simulink model "MainSim"  (R2025a)
settings: Solver=VariableStepAuto  StartTime=0.0  StopTime=110  MaxStep=0.01  RelTol=1e-3
undefined symbols (not defined in the file): bref, cref, g, inertia, m, m_carriage
libraries: fl_lib x79, nesl_utility x32, simulink_extras x9, sdl_lib x4, aerolibobsolete x2, ee_lib x2, slpidlib x2, aerolibadyn x1, matrix_library x1, aerolibatmos2 x1, aerolibwind2 x1, aerolibanim x1
(part 3 of 5)

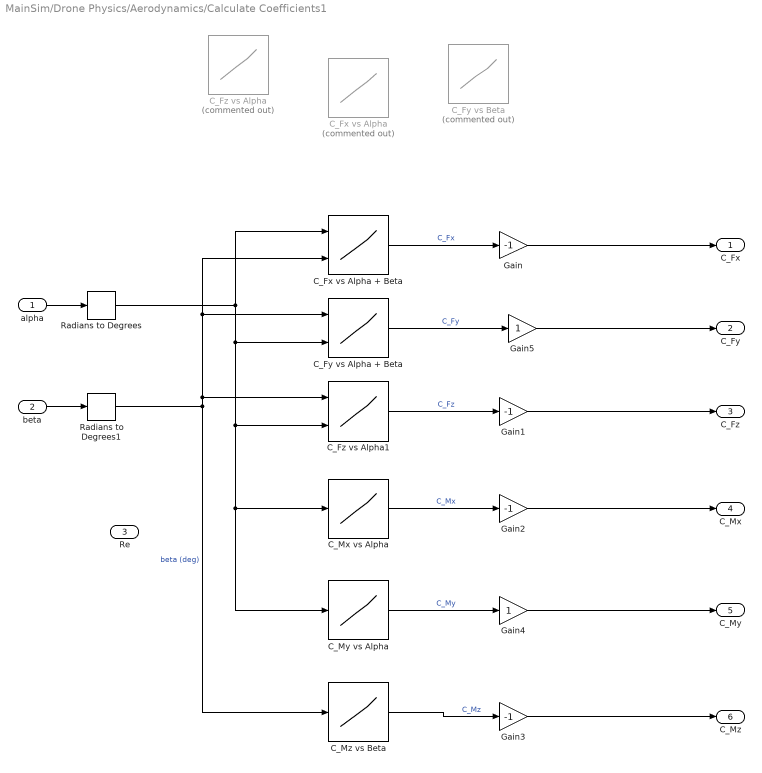
== system MainSim/Drone Physics/Aerodynamics/Calculate Coefficients1 ==
  alpha : Inport
  beta : Inport  Port=2
  Re : Inport  Port=3
  C_Fx vs Alpha : Lookup_n-D  Commented=on  NumberOfTableDimensions=1  BreakpointsForDimension1=[-30;-24;-18;-12;-6;-1;1;6;12;18;24;30]  Table=[-0.8477543;-0.5413928;-0.2881651;-0.0989454;0.01802407;0.06513188;0.06513188;0.01802407;-0.0989454;-0.2881651;-0.5413928;-0.8477543]  InternalRulePriority=Speed  RndMeth=Simplest
  C_Fx vs Alpha + Beta : Lookup_n-D  BreakpointsForDimension1=[-20;-18;-16;-14;-12;-10;-8;-6;-4;-2;0;2;4;6;8;10;12;14;16;18;20]  BreakpointsForDimension2=[-20;-18;-16;-14;-12;-10;-8;-6;-4;-2;0;2;4;6;8;10;12;14;16;18;20]  Table=[-0.614358525 -0.552468628 -0.496975921 -0.447963654 -0.405402727 -0.369395384 -0.339949206 -0.317050883 -0.300725231 -0.290929286 -0.287706806 -0.290929286 -0.300725231 -0.317050883 -0.339949206 -0.369395384 -0.405402727 -0.447963654 -0.496975921 -0.552468628 -0.614358525;-0.551607695 -0.489072561 -0.432947474 -0.383480964 -0.340566675 -0.304256004 -0.274532451 -0.251406615 -0.234924884 -0.22504748 -0.221789714 -0.22504748 -0.234924884 -0.251406615 -0.274532451 -0.304256004 -0.340566675 -0.383480964 -0.432947474 -0.489072561 -0.551607695;-0.495317375 -0.432168752 -0.375672546 -0.325789814 -0.282533426 -0.245910781 -0.215944692 -0.192643052 -0.176018972 -0.16606146 -0.162782923 -0.16606146 -0.176018972 -0.192643052 -0.215944692 -0.245910781 -0.282533426 -0.325789814 -0.375672546 -0.432168752 -0.495317375;-0.445552671 -0.382005906 -0.325091967 -0.274839973 -0.231277677 -0.194399013 -0.164233169 -0.140770136 -0.124023873 -0.113987385 -0.110686666 -0.113987385 -0.124023873 -0.140770136 -0.164233169 -0.194399013 -0.231277677 -0.274839973 -0.325091967 -0.382005906 -0.445552671;-0.40242558 -0.338476077 -0.281206427 -0.230652283 -0.186829361 -0.149732411 -0.119392246 -0.095788054 -0.07893594700000001 -0.06885042800000001 -0.065514827 -0.06885042800000001 -0.07893594700000001 -0.095788054 -0.119392246 -0.149732411 -0.186829361 -0.230652283 -0.281206427 -0.338476077 -0.40242558;-0.365919483 -0.301631518 -0.244075562 -0.193256152 -0.149204048 -0.111925303 -0.081432692 -0.057717714 -0.040804565 -0.030673395 -0.027308541 -0.030673395 -0.040804565 -0.057717714 -0.081432692 -0.111925303 -0.149204048 -0.193256152 -0.244075562 -0.301631518 -0.365919483;-0.336041187 -0.271485221 -0.213680187 -0.162651643 -0.118419577 -0.080997789 -0.050375282 -0.026586135 -0.009594434000000001 0.000582762 0.003952354 0.000582762 -0.009594434000000001 -0.026586135 -0.050375282 -0.080997789 -0.118419577 -0.162651643 -0.213680187 -0.271485221 -0.336041187;-0.312780091 -0.248011918 -0.190027999 -0.138840895 -0.094478059 -0.056945223 -0.026238136 -0.00236637 0.014675995 0.024884562 0.028280614 0.024884562 0.014675995 -0.00236637 -0.026238136 -0.056945223 -0.094478059 -0.138840895 -0.190027999 -0.248011918 -0.312780091;-0.296181899 -0.231254063 -0.173135414 -0.121838779 -0.077382601 -0.039773232 -0.008997109 0.014930056 0.032010963 0.042247716 0.045634461 0.042247716 0.032010963 0.014930056 -0.008997109 -0.039773232 -0.077382601 -0.121838779 -0.173135414 -0.231254063 -0.296181899;-0.28623251 -0.221218221 -0.163015263 -0.11165277 -0.06713633400000001 -0.029480985 0.001340551 0.025308445 0.042403284 0.052657162 0.0560561 0.052657162 0.042403284 0.025308445 0.001340551 -0.029480985 -0.06713633400000001 -0.11165277 -0.163015263 -0.221218221 -0.28623251;-0.217886618 -0.217886618 -0.15966593 -0.108275856 -0.06373363 -0.026060496 0.004776964 0.028752083 0.045865859 0.056122123 0.059524976 0.056122123 0.045865859 0.028752083 0.004776964 -0.026060496 -0.06373363 -0.108275856 -0.15966593 -0.217886618 -0.217886618;-0.28623251 -0.221218221 -0.163015263 -0.11165277 -0.06713633400000001 -0.029480985 0.001340551 0.025308445 0.042403284 0.052657162 0.0560561 0.052657162 0.042403284 0.025308445 0.001340551 -0.029480985 -0.06713633400000001 -0.11165277 -0.163015263 -0.221218221 -0.28623251;-0.296181899 -0.231254063 -0.173135414 -0.121838779 -0.077382601 -0.039773232 -0.008997109 0.014930056 0.032010963 0.042247716 0.045634461 0.042247716 0.032010963 0.014930056 -0.008997109 -0.039773232 -0.077382601 -0.121838779 -0.173135414 -0.231254063 -0.296181899;-0.312780091 -0.248011918 -0.190027999 -0.138840895 -0.094478059 -0.056945223 -0.026238136 -0.00236637 0.014675995 0.024884562 0.028280614 0.024884562 0.014675995 -0.00236637 -0.026238136 -0.056945223 -0.094478059 -0.138840895 -0.190027999 -0.248011918 -0.312780091;-0.336041187 -0.271485221 -0.213680187 -0.162651643 -0.118419577 -0.080997789 -0.050375282 -0.026586135 -0.009594434000000001 0.000582762 0.003952354 0.000582762 ...(+1790 chars)]  InternalRulePriority=Speed  RndMeth=Simplest
      settings: InputPortMap=u0,u1
  C_Fy vs Alpha + Beta : Lookup_n-D  BreakpointsForDimension1=[-20;-18;-16;-14;-12;-10;-8;-6;-4;-2;0;2;4;6;8;10;12;14;16;18;20]  BreakpointsForDimension2=[-20;-18;-16;-14;-12;-10;-8;-6;-4;-2;0;2;4;6;8;10;12;14;16;18;20]  Table=[1.66195002 1.66627986 1.67002882 1.67327787 1.67699593 1.67878935 1.68047312 1.6822726 1.68322903 1.68369328 1.68391417 1.68369328 1.68322903 1.6822726 1.68047312 1.67878935 1.67699593 1.67327787 1.67002882 1.66627986 1.66195002;1.50492698 1.50889275 1.51325693 1.51613012 1.5186286 1.52053747 1.52211226 1.5230983 1.52411176 1.52465096 1.52475781 1.52465096 1.52411176 1.5230983 1.52211226 1.52053747 1.5186286 1.51613012 1.51325693 1.50889275 1.50492698;1.3449861 1.34965961 1.35276007 1.3553714 1.35760143 1.35922371 1.36072185 1.36169609 1.36221375 1.36277715 1.36305841 1.36277715 1.36221375 1.36169609 1.36072185 1.35922371 1.35760143 1.3553714 1.35276007 1.34965961 1.3449861;1.18364169 1.18651461 1.18940186 1.1919222 1.19406535 1.19564439 1.19670122 1.1974075 1.19789162 1.19833631 1.19861313 1.19833631 1.19789162 1.1974075 1.19670122 1.19564439 1.19406535 1.1919222 1.18940186 1.18651461 1.18364169;1.01863302 1.02137777 1.02382367 1.02623563 1.02802096 1.0291959 1.03039533 1.03091195 1.03143754 1.03171442 1.03166744 1.03171442 1.03143754 1.03091195 1.03039533 1.0291959 1.02802096 1.02623563 1.02382367 1.02137777 1.01863302;0.85160149 0.854263182 0.856389587 0.85839774 0.860011937 0.861116685 0.8621121899999999 0.862633629 0.862917173 0.863469112 0.863402469 0.863469112 0.862917173 0.862633629 0.8621121899999999 0.861116685 0.860011937 0.85839774 0.856389587 0.854263182 0.85160149;0.683145201 0.6854003870000001 0.687448977 0.689359965 0.690391124 0.691442623 0.691573132 0.692106162 0.69270664 0.693189344 0.693075696 0.693189344 0.69270664 0.692106162 0.691573132 0.691442623 0.690391124 0.689359965 0.687448977 0.6854003870000001 0.683145201;0.513680454 0.515516389 0.51700176 0.518329265 0.519440831 0.520452311 0.51978407 0.520476755 0.521151285 0.521719227 0.521682795 0.521719227 0.521151285 0.520476755 0.51978407 0.520452311 0.519440831 0.518329265 0.51700176 0.515516389 0.513680454;0.342987019 0.344595797 0.345799223 0.346543215 0.347632555 0.346986164 0.34735697 0.34791355 0.348772052 0.349005705 0.348832678 0.349005705 0.348772052 0.34791355 0.34735697 0.346986164 0.347632555 0.346543215 0.345799223 0.344595797 0.342987019;0.171657723 0.172615507 0.173702671 0.174327657 0.174967248 0.1739672 0.1742629 0.174639945 0.175310283 0.175362274 0.175197751 0.175362274 0.175310283 0.174639945 0.1742629 0.1739672 0.174967248 0.174327657 0.173702671 0.172615507 0.171657723;-0.000932729 -0.000932729 -0.001325927 -0.001861466 -0.002017838 -0.000728378 -0.000836194 -0.001162275 -0.00131784 -0.001113439 -0.00023498 -0.001113439 -0.00131784 -0.001162275 -0.000836194 -0.000728378 -0.002017838 -0.001861466 -0.001325927 -0.000932729 -0.000932729;-0.171657723 -0.172615507 -0.173702671 -0.174327657 -0.174967248 -0.1739672 -0.1742629 -0.174639945 -0.175310283 -0.175362274 -0.175197751 -0.175362274 -0.175310283 -0.174639945 -0.1742629 -0.1739672 -0.174967248 -0.174327657 -0.173702671 -0.172615507 -0.171657723;-0.342987019 -0.344595797 -0.345799223 -0.346543215 -0.347632555 -0.346986164 -0.34735697 -0.34791355 -0.348772052 -0.349005705 -0.348832678 -0.349005705 -0.348772052 -0.34791355 -0.34735697 -0.346986164 -0.347632555 -0.346543215 -0.345799223 -0.344595797 -0.342987019;-0.513680454 -0.515516389 -0.51700176 -0.518329265 -0.519440831 -0.520452311 -0.51978407 -0.520476755 -0.521151285 -0.521719227 -0.521682795 -0.521719227 -0.521151285 -0.520476755 -0.51978407 -0.520452311 -0.519440831 -0.518329265 -0.51700176 -0.515516389 -0.513680454;-0.683145201 -0.6854003870000001 -0.687448977 -0.689359965 -0.690391124 -0.691442623 -0.691573132 -0.692106162 -0.69270664 -0.693189344 -0.693075696 -0.693189344 -0.69270664 -0.692106162 -0.691573132 -0.691442623 -0.690391124 -0.689359965 -0.687448977 -0.6854003870000001 -0.683145201;-0.85160149 -0.854263182 -0.856389587 -0.85839774 -0.860011937 -0.861116685 -0.8621121899999999 -0.862633629 -0.862917173 -0.863469112 -0.863402469 -0.863469112 -0.862917173 -0.862633629 -0.8621121899999999 -0.861116685 -0.860011937 ...(+1294 chars)]  ExtrapMethod=Clip  InternalRulePriority=Speed  RndMeth=Simplest
      settings: InputPortMap=u0,u1
  C_Fy vs Beta : Lookup_n-D  Commented=on  NumberOfTableDimensions=1  BreakpointsForDimension1=[-30;-24;-18;-12;-6;-1;1;6;12;16;20;25;30;35;40;45;50;60;70;90]  Table=[-2.6204513;-2.2457427000000001;-1.7747444000000001;-1.2274444;-0.62725549999999997;-0.079830300000000007;0.079830310000000002;0.62725547000000004;1.22744436;1.6399999999999999;1.8999999999999999;1.1000000000000001;1.05;1;1;1;0.90000000000000002;0.5;0.29999999999999999;0]  ExtrapMethod=Clip  InternalRulePriority=Speed  RndMeth=Simplest
  C_Fz vs Alpha : Lookup_n-D  Commented=on  NumberOfTableDimensions=1  BreakpointsForDimension1=[-30;-24;-18;-12;-6;-1;1;6;12;16;20;25;30;35;40;45;50;60;70;90]  Table=[-2.6204513;-2.2457427000000001;-1.7747444000000001;-1.2274444;-0.62725549999999997;-0.079830300000000007;0.079830310000000002;0.62725547000000004;1.22744436;1.6399999999999999;1.8999999999999999;1.1000000000000001;1.05;1;1;1;0.90000000000000002;0.5;0.29999999999999999;0]  ExtrapMethod=Clip  InternalRulePriority=Speed  RndMeth=Simplest
  C_Fz vs Alpha1 : Lookup_n-D  BreakpointsForDimension1=[-20;-18;-16;-14;-12;-10;-8;-6;-4;-2;0;2;4;6;8;10;12;14;16;18;20]  BreakpointsForDimension2=[-20;-18;-16;-14;-12;-10;-8;-6;-4;-2;0;2;4;6;8;10;12;14;16;18;20]  Table=[-1.55009948 -1.40370092 -1.25462317 -1.10283778 -0.949156016 -0.7935119390000001 -0.636432656 -0.477775325 -0.318386645 -0.158573043 -0.001764467 0.158573043 0.318386645 0.477775325 0.636432656 0.7935119390000001 0.949156016 1.10283778 1.25462317 1.40370092 1.55009948;-1.57242746 -1.42392316 -1.27291412 -1.11875403 -0.962481446 -0.804477256 -0.644911779 -0.484281407 -0.322789156 -0.160769242 -0.002307224 0.160769242 0.322789156 0.484281407 0.644911779 0.804477256 0.962481446 1.11875403 1.27291412 1.42392316 1.57242746;-1.59261224 -1.44260011 -1.28893724 -1.13291699 -0.974830801 -0.814870303 -0.653020572 -0.490346781 -0.32667547 -0.162246361 -0.002565448 0.162246361 0.32667547 0.490346781 0.653020572 0.814870303 0.974830801 1.13291699 1.28893724 1.44260011 1.59261224;-1.61091112 -1.45846414 -1.30317135 -1.14538593 -0.985506982 -0.823595326 -0.660151009 -0.495668672 -0.330141696 -0.163784707 -0.002650902 0.163784707 0.330141696 0.495668672 0.660151009 0.823595326 0.985506982 1.14538593 1.30317135 1.45846414 1.61091112;-1.62580438 -1.47213576 -1.31538824 -1.15589718 -0.994589284 -0.831455457 -0.666675567 -0.500644752 -0.333363011 -0.165359101 -0.002762659 0.165359101 0.333363011 0.500644752 0.666675567 0.831455457 0.994589284 1.15589718 1.31538824 1.47213576 1.62580438;-1.6394278 -1.48424315 -1.32634589 -1.16560392 -1.00278587 -0.838339093 -0.672240555 -0.50496377 -0.33688758 -0.167824235 -0.002242482 0.167824235 0.33688758 0.50496377 0.672240555 0.838339093 1.00278587 1.16560392 1.32634589 1.48424315 1.6394278;-1.65045554 -1.49444956 -1.33532388 -1.17333149 -1.00982805 -0.844082802 -0.677467162 -0.509090802 -0.339530444 -0.169133362 -0.001356052 0.169133362 0.339530444 0.509090802 0.677467162 0.844082802 1.00982805 1.17333149 1.33532388 1.49444956 1.65045554;-1.65862927 -1.50181487 -1.34209337 -1.1796587 -1.01530082 -0.84885035 -0.681215192 -0.5120618220000001 -0.341559843 -0.170311443 -0.00127523 0.170311443 0.341559843 0.5120618220000001 0.681215192 0.84885035 1.01530082 1.1796587 1.34209337 1.50181487 1.65862927;-1.66490423 -1.507349 -1.34699511 -1.18436577 -1.01945538 -0.853198533 -0.684158833 -0.514192369 -0.343166457 -0.17152109 -0.000870461 0.17152109 0.343166457 0.514192369 0.684158833 0.853198533 1.01945538 1.18436577 1.34699511 1.507349 1.66490423;-1.66880981 -1.51086475 -1.35022719 -1.18731356 -1.02212124 -0.855586551 -0.686012383 -0.515670089 -0.344273714 -0.172312963 -0.000435662 0.172312963 0.344273714 0.515670089 0.686012383 0.855586551 1.02212124 1.18731356 1.35022719 1.51086475 1.66880981;-1.5118782 -1.5118782 -1.35139134 -1.18847636 -1.02316789 -0.856422645 -0.686794229 -0.516544166 -0.344670939 -0.172784026 -4.74e-05 0.172784026 0.344670939 0.516544166 0.686794229 0.856422645 1.02316789 1.18847636 1.35139134 1.5118782 1.5118782;-1.66880981 -1.51086475 -1.35022719 -1.18731356 -1.02212124 -0.855586551 -0.686012383 -0.515670089 -0.344273714 -0.172312963 -0.000435662 0.172312963 0.344273714 0.515670089 0.686012383 0.855586551 1.02212124 1.18731356 1.35022719 1.51086475 1.66880981;-1.66490423 -1.507349 -1.34699511 -1.18436577 -1.01945538 -0.853198533 -0.684158833 -0.514192369 -0.343166457 -0.17152109 -0.000870461 0.17152109 0.343166457 0.514192369 0.684158833 0.853198533 1.01945538 1.18436577 1.34699511 1.507349 1.66490423;-1.65862927 -1.50181487 -1.34209337 -1.1796587 -1.01530082 -0.84885035 -0.681215192 -0.5120618220000001 -0.341559843 -0.170311443 -0.00127523 0.170311443 0.341559843 0.5120618220000001 0.681215192 0.84885035 1.01530082 1.1796587 1.34209337 1.50181487 1.65862927;-1.65045554 -1.49444956 -1.33532388 -1.17333149 -1.00982805 -0.844082802 -0.677467162 -0.509090802 -0.339530444 -0.169133362 -0.001356052 0.169133362 0.339530444 0.509090802 0.677467162 0.844082802 1.00982805 1.17333149 1.33532388 1.49444956 1.65045554;-1.6394278 -1.48424315 -1.32634589 -1.16560392 -1.00278587 -0.838339093 -0.672240555 -0.50496377 -0.33688758 -0.167824235 -0.002242482 0.167824235 0.33688758 0.50496377 0.672240555 ...(+1353 chars)]  ExtrapMethod=Clip  InternalRulePriority=Speed  RndMeth=Simplest
      settings: InputPortMap=u0,u1
  C_Mx vs Alpha : Lookup_n-D  NumberOfTableDimensions=1  BreakpointsForDimension1=[-15;-11.25;-7.5;-3.75;-2;-1.7777780000000001;-1.5555559999999999;-1.3333330000000001;-1.111111;-0.88888900000000004;-0.66666700000000001;-0.44444400000000001;-0.222222;0;0.222222;0.44444400000000001;0.66666700000000001;0.88888900000000004;1.111111;1.3333330000000001;1.5555559999999999;1.7777780000000001;2;3.75;7.5;11.25;15]  Table=[8.330000000000001e-05;4.3e-05;1.83e-05;3.47e-06;5.9e-07;3.8e-07;2.58e-07;1.93e-07;1.74e-07;1.53e-07;1.57e-07;2e-07;2.8e-07;-3.94e-07;-2.8e-07;-2e-07;-1.57e-07;-1.53e-07;-1.74e-07;-1.93e-07;-2.58e-07;-3.8e-07;-5.9e-07;-3.47e-06;-1.83e-05;-4.3e-05;-8.330000000000001e-05]  InternalRulePriority=Speed  RndMeth=Simplest
  C_My vs Alpha : Lookup_n-D  NumberOfTableDimensions=1  BreakpointsForDimension1=[-30;-24;-18;-12;-6;-1;1;6;12;18;24;30]  Table=[0.63433291;0.54398872;0.43026972;0.29781773;0.15227498;0.01398048;-0.0139805;-0.152275;-0.2978177;-0.4302697;-0.5439887;-0.6343329]  InternalRulePriority=Speed  RndMeth=Simplest
  C_Mz vs Beta : Lookup_n-D  NumberOfTableDimensions=1  BreakpointsForDimension1=[-30;-24;-18;-12;-6;-1;1;6;12;18;24;30]  Table=[0.63433291;0.54398872;0.43026972;0.29781773;0.15227498;0.01398048;-0.0139805;-0.152275;-0.2978177;-0.4302697;-0.5439887;-0.6343329]  InternalRulePriority=Speed  RndMeth=Simplest
  Gain{,1..3} (4 alike) : Gain  Gain=-1
  Gain4 : Gain
  Gain5 : Gain
  Radians to Degrees : simulink_extras/Transformations/Radians to Degrees
  Radians to Degrees1 : simulink_extras/Transformations/Radians to Degrees
  C_Fx : Outport
  C_Fy : Outport  Port=2
  C_Fz : Outport  Port=3
  C_Mx : Outport  Port=4
  C_My : Outport  Port=5
  C_Mz : Outport  Port=6
  wires:
  Gain5/1 -> C_Fy/1
  Gain4/1 -> C_My/1
  Gain3/1 -> C_Mz/1
  Gain2/1 -> C_Mx/1
  Gain1/1 -> C_Fz/1
  Gain/1 -> C_Fx/1
  Radians to Degrees1/1 -> C_Fz vs Alpha1/1, C_Fy vs Alpha + Beta/1, C_Fx vs Alpha + Beta/2, C_Mz vs Beta/1  "beta (deg)"
  Radians to Degrees/1 -> C_Fx vs Alpha + Beta/1, C_Fy vs Alpha + Beta/2, C_Fz vs Alpha1/2, C_Mx vs Alpha/1, C_My vs Alpha/1
  C_Mz vs Beta/1 -> Gain3/1  "C_Mz"
  C_My vs Alpha/1 -> Gain4/1  "C_My"
  C_Mx vs Alpha/1 -> Gain2/1  "C_Mx"
  beta/1 -> Radians to Degrees1/1
  alpha/1 -> Radians to Degrees/1
  C_Fy vs Alpha + Beta/1 -> Gain5/1  "C_Fy"
  C_Fz vs Alpha1/1 -> Gain1/1  "C_Fz"
  C_Fx vs Alpha + Beta/1 -> Gain/1  "C_Fx"

== system MainSim/Drone Physics/EoM/Combine Forces & Moments ==
  Aerodynamics : Inport
  Gravity : Inport  Port=2
  Propulsion : Inport  Port=3
  CG : Inport  Port=4
  Add : Sum  Inputs=+++
  Add1 : Sum  Inputs=++++++
  Bus Selector : BusSelector  OutputSignals=F_B,M_B,S_B
  Bus Selector1 : BusSelector  OutputSignals=F_B,M_B,S_B
  Bus Selector2 : BusSelector  OutputSignals=F_B,M_B
  Cross Product : matrix_library/Cross Product
  Gain : Gain  Gain=1/cref
  Subtract : Sum  Inputs=+-
  Terminator : Terminator
  F_B' : Outport
  M_B' : Outport  Port=2
  wires:
  Aerodynamics/1 -> Bus Selector/1
  Gravity/1 -> Bus Selector1/1
  Add/1 -> F_B'/1  "F_B'"
  Add1/1 -> M_B'/1
  Bus Selector/1 -> Cross Product/2, Add/1  "<F_B>"
  Bus Selector1/1 -> Add/2  "<F_B>"
  Bus Selector/2 -> Add1/1  "<M_B>"
  Bus Selector/3 -> Subtract/1  "<S_B>"
  Subtract/1 -> Cross Product/1
  Cross Product/1 -> Add1/2
  Gain/1 -> Terminator/1  "CG/C"
  CG/1 -> Gain/1, Subtract/2
  Propulsion/1 -> Bus Selector2/1
  Bus Selector2/2 -> Add1/3  "<M_B>"
  Bus Selector2/1 -> Add/3  "<F_B>"

== system MainSim/Drone Physics/EoM/Direction Cosine Matrix Calculation ==
  Eul_BL : Inport
  Demux : Demux  Outputs=3
  Ground : Ground
  Rotation Angles to Direction Cosine Matrix : Angle2Dcm
      settings: AttributesFormatString=Rotation Order: %<rotationOrder>
  Terminator : Terminator
  Terminator1 : Terminator
  Transpose : Math  Operator=transpose
  Vector Concatenate : Concatenate  NumInputs=3
  DCM_B'B : Outport
  DCM_BB' : Outport  Port=2
  wires:
  Demux/3 -> Terminator1/1
  Transpose/1 -> DCM_B'B/1  "DCM_B'B"
  Vector Concatenate/1 -> Rotation Angles to Direction Cosine Matrix/1
  Rotation Angles to Direction Cosine Matrix/1 -> DCM_BB'/1, Transpose/1  "DCM_BB'"
  Ground/1 -> Vector Concatenate/2, Vector Concatenate/1
  Demux/2 -> Terminator/1
  Demux/1 -> Vector Concatenate/3
  Eul_BL/1 -> Demux/1

== system MainSim/Drone Physics/EoM/Ground Detect Trigger - Termination ==
  X_BE_E : Inport
  Ground Level : Constant  Value=ground_level
  Relational Operator : RelationalOperator  Operator=>  OutDataTypeStr=boolean  RndMeth=Simplest  InputSameDT=off
  Selector : Selector  InputPortWidth=3  IndexOptions=Index vector (dialog)  Indices=[3]  OutputSizes=1
  Stop Simulation : Stop
  wires:
  Relational Operator/1 -> Stop Simulation/1
  Ground Level/1 -> Relational Operator/2
  X_BE_E/1 -> Selector/1
  Selector/1 -> Relational Operator/1

== system MainSim/Drone Physics/EoM/Running Avg ==
  u : Inport
  MATLAB Function : MATLAB Function  TreatAsAtomicUnit=on
  Out1 : Outport
  wires:
  u/1 -> MATLAB Function/1(u)
  MATLAB Function/1(y) -> Out1/1

== system MainSim/Drone Physics/EoM/Running Avg1 ==
  u : Inport
  MATLAB Function : MATLAB Function  TreatAsAtomicUnit=on
  Out1 : Outport
  wires:
  u/1 -> MATLAB Function/1(u)
  MATLAB Function/1(y) -> Out1/1

== system MainSim/Drone Physics/EoM/Running Avg2 ==
  u : Inport
  MATLAB Function : MATLAB Function  TreatAsAtomicUnit=on
  Out1 : Outport
  wires:
  u/1 -> MATLAB Function/1(u)
  MATLAB Function/1(y) -> Out1/1

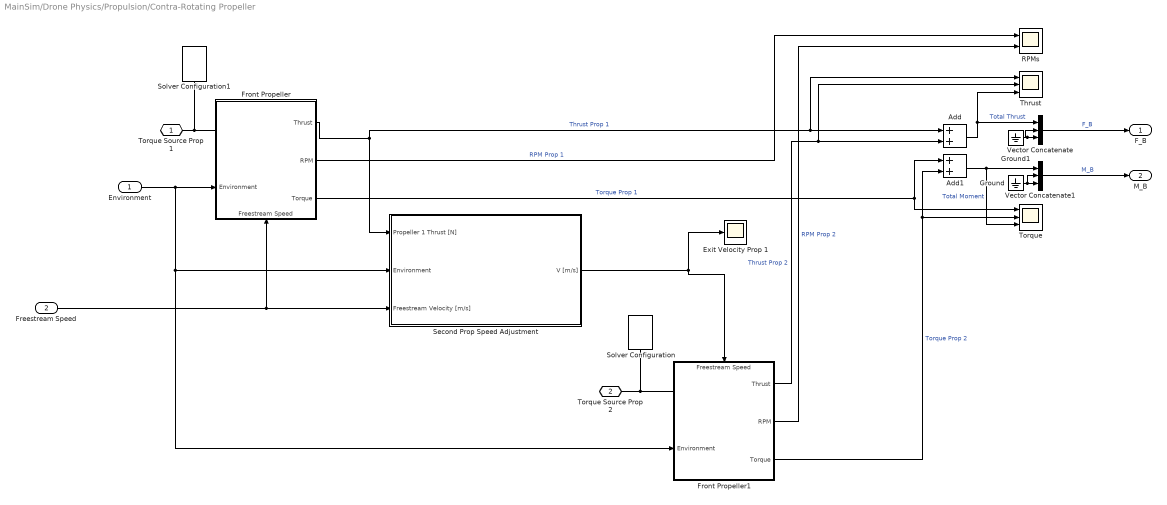
== system MainSim/Drone Physics/Propulsion/Contra-Rotating Propeller ==
  Environment : Inport
  Freestream Speed : Inport  Port=2
  Add : Sum
  Add1 : Sum
  Exit Velocity Prop 1 : Scope
      settings: ActiveDisplayYMinimum=-0.56468572092452329  ActiveDisplayYMaximum=5.0821714883207108  DataLoggingVariableName=ScopeData5
  Front Propeller : Subsystem
      settings: PortSchema="{\"entries\":[{\"content\":{\"sides\":[{\"content\":{\"connectorIds\":[\"LConn1\",\"In1\"]},\"type\":\"ConnectorPlacement.EquallySpacedRectSide\",\"uuid\":\"73d37dfa-c503-43f9-9596-b5e45f2bb291\"},{\"content\":{\"connectorIds\":[\"Out1\",\"Out2\",\"Out3\"],\"side\":\"RIGHT\"},\"type\":\"ConnectorPlacement.EquallySpacedRectSide\",\"uuid\":\"3674c389-2fff-4609-bdea-497312b626f0\"},{\"content\":{\"side\":\"TOP\"},\"type\":\"ConnectorPlacement.EquallySpacedRectSide\",\"uuid\":\"4ddff869-abc5-41ea-b654-b1a87db3aebf\"},{\"content\":{\"connectorIds\":[\"In2\"],\"side\":\"BOTTOM\"},\"type\":\"ConnectorPlacement.EquallySpacedRectSide\",\"uuid\":\"b118b9bb-d518-4709-95e5-457ee8be32dc\"}]},\"type\":\"ConnectorPlacement.EquallySpacedConnector\",\"uuid\":\"ef4d0754-f307-49aa-90cb-f59c4d3f0201\"}],\"packageUris\":[\"http://schema.mathworks.com/mf0/Connector/R2020b\"],\"version\":\"1.0\"}"
  Front Propeller1 : Subsystem
      settings: PortSchema="{\"entries\":[{\"content\":{\"sides\":[{\"content\":{\"connectorIds\":[\"LConn1\",\"In1\"]},\"type\":\"ConnectorPlacement.EquallySpacedRectSide\",\"uuid\":\"73d37dfa-c503-43f9-9596-b5e45f2bb291\"},{\"content\":{\"connectorIds\":[\"Out1\",\"Out2\",\"Out3\"],\"side\":\"RIGHT\"},\"type\":\"ConnectorPlacement.EquallySpacedRectSide\",\"uuid\":\"3674c389-2fff-4609-bdea-497312b626f0\"},{\"content\":{\"connectorIds\":[\"In2\"],\"side\":\"TOP\"},\"type\":\"ConnectorPlacement.EquallySpacedRectSide\",\"uuid\":\"4ddff869-abc5-41ea-b654-b1a87db3aebf\"}]},\"type\":\"ConnectorPlacement.EquallySpacedConnector\",\"uuid\":\"ef4d0754-f307-49aa-90cb-f59c4d3f0201\"}],\"packageUris\":[\"http://schema.mathworks.com/mf0/Connector/R2020b\"],\"version\":\"1.0\"}"
  Ground : Ground
  Ground1 : Ground
  RPMs : Scope  NumInputPorts=2
      settings: ActiveDisplayYMinimum=-11573.712044991189  ActiveDisplayYMaximum=11896.938453382989  DataLoggingVariableName=ScopeData4
  Second Prop Speed Adjustment : Subsystem
  Solver Configuration : nesl_utility/Solver Configuration  PhysicalDomain=network_engine_domain  SubClassName=solver  LeftPortType=input  RightPortType=generic  Tones=[]  Harmonics=[]  SimulateNoise=off  Profile=off  UseLocalSampling=off  EnableSwitchedLinearOptims=on  FrequencyDomain=off  UseCCode=off  RelTol=0.001  AbsTol=0.001  MinStep=1e-09  ToWorkspace=off  RevertToSquareIcSolve=off  NumHomotopyIterations=100  PhasorMode=off  PhasorModeNumHarmonics=1  ConsistencySolver=NEWTON_XTOL_AFTER_FTOL  IndexReductionMethod=DerivativeReplacement  DoDC=off  ResidualTolerance=1e-09  ConsistencyTolSource=GLOBAL  ConsistencyAbsTol=0.001  ConsistencyRelTol=0.001  ConsistencyTolFactor=0.001  UseLocalSolver=off  LocalSolverChoice=NE_BACKWARD_EULER_ADVANCER  ResolveIndetEquations=on  FunctionEvalNumThread=1  LocalSolverSampleTime=0.001  DoFixedCost=off  MaxNonlinIter=3  MaxModeIter=2  ComputeImpulses=off  ImpulseIterations=2  LinearAlgebra=auto  LinearAlgebraNumThread=0  EquationFormulation=NE_TIME_EF  DelaysMemoryBudget=1024  AutomaticFiltering=on  FilteringTimeConstant=0.001  PartitionStorageMethod=AS_NEEDED  PartitionMemoryBudget=1024  PartitionMethod=ROBUST  MultibodyUseLocalSolver=off  MultibodyLocalSolverChoice=ODE1  MultibodyLocalSolverSampleTime=0.001
  Solver Configuration1 : nesl_utility/Solver Configuration  PhysicalDomain=network_engine_domain  SubClassName=solver  LeftPortType=input  RightPortType=generic  Tones=[]  Harmonics=[]  SimulateNoise=off  Profile=off  UseLocalSampling=off  EnableSwitchedLinearOptims=on  FrequencyDomain=off  UseCCode=off  RelTol=0.001  AbsTol=0.001  MinStep=1e-09  ToWorkspace=off  RevertToSquareIcSolve=off  NumHomotopyIterations=100  PhasorMode=off  PhasorModeNumHarmonics=1  ConsistencySolver=NEWTON_XTOL_AFTER_FTOL  IndexReductionMethod=DerivativeReplacement  DoDC=off  ResidualTolerance=1e-09  ConsistencyTolSource=GLOBAL  ConsistencyAbsTol=0.001  ConsistencyRelTol=0.001  ConsistencyTolFactor=0.001  UseLocalSolver=off  LocalSolverChoice=NE_BACKWARD_EULER_ADVANCER  ResolveIndetEquations=on  FunctionEvalNumThread=1  LocalSolverSampleTime=0.001  DoFixedCost=off  MaxNonlinIter=3  MaxModeIter=2  ComputeImpulses=off  ImpulseIterations=2  LinearAlgebra=auto  LinearAlgebraNumThread=0  EquationFormulation=NE_TIME_EF  DelaysMemoryBudget=1024  AutomaticFiltering=on  FilteringTimeConstant=0.001  PartitionStorageMethod=AS_NEEDED  PartitionMemoryBudget=1024  PartitionMethod=ROBUST  MultibodyUseLocalSolver=off  MultibodyLocalSolverChoice=ODE1  MultibodyLocalSolverSampleTime=0.001
  Thrust : Scope  NumInputPorts=3
      settings: ActiveDisplayYMinimum=-0.51224883046910774  ActiveDisplayYMaximum=4.1562383451302329
  Torque : Scope  NumInputPorts=3
      settings: ActiveDisplayYMinimum=-0.0788123767098801  ActiveDisplayYMaximum=0.078815374675042418  DataLoggingVariableName=ScopeData6
  Vector Concatenate : Concatenate  NumInputs=3
  Vector Concatenate1 : Concatenate  NumInputs=3
  Torque Source Prop 1 : PMIOPort  Side=Left
  Torque Source Prop 2 : PMIOPort  Port=2  Side=Left
  F_B : Outport
  M_B : Outport  Port=2
  wires:
  Add/1 -> Thrust/3, Vector Concatenate/1  "Total Thrust"
  Freestream Speed/1 -> Front Propeller/2(Freestream Speed), Second Prop Speed Adjustment/3(Freestream Velocity [m/s])
  Ground/1 -> Vector Concatenate1/2, Vector Concatenate1/3
  Vector Concatenate/1 -> F_B/1  "F_B"
  Front Propeller1/1(Thrust) -> Thrust/2, Add/2  "Thrust Prop 2"
  Front Propeller/3(Torque) -> Torque/1, Add1/1  "Torque Prop 1"
  Ground1/1 -> Vector Concatenate/2, Vector Concatenate/3
  Front Propeller1/3(Torque) -> Add1/2, Torque/2  "Torque Prop 2"
  Front Propeller1/2(RPM) -> RPMs/2  "RPM Prop 2"
  Vector Concatenate1/1 -> M_B/1  "M_B"
  Environment/1 -> Front Propeller1/1(Environment), Second Prop Speed Adjustment/2(Environment), Front Propeller/1(Environment)
  Front Propeller/2(RPM) -> RPMs/1  "RPM Prop 1"
  Second Prop Speed Adjustment/1(V [m/s]) -> Front Propeller1/2(Freestream Speed), Exit Velocity Prop 1/1
  Add1/1 -> Torque/3, Vector Concatenate1/1  "Total Moment"
  Front Propeller/1(Thrust) -> Thrust/1, Add/1, Second Prop Speed Adjustment/1(Propeller 1 Thrust [N])  "Thrust Prop 1"
  connections:
  Torque Source Prop 2/RConn1 -- Front Propeller1/LConn1 -- Solver Configuration/RConn1
  Torque Source Prop 1/RConn1 -- Solver Configuration1/RConn1 -- Front Propeller/LConn1

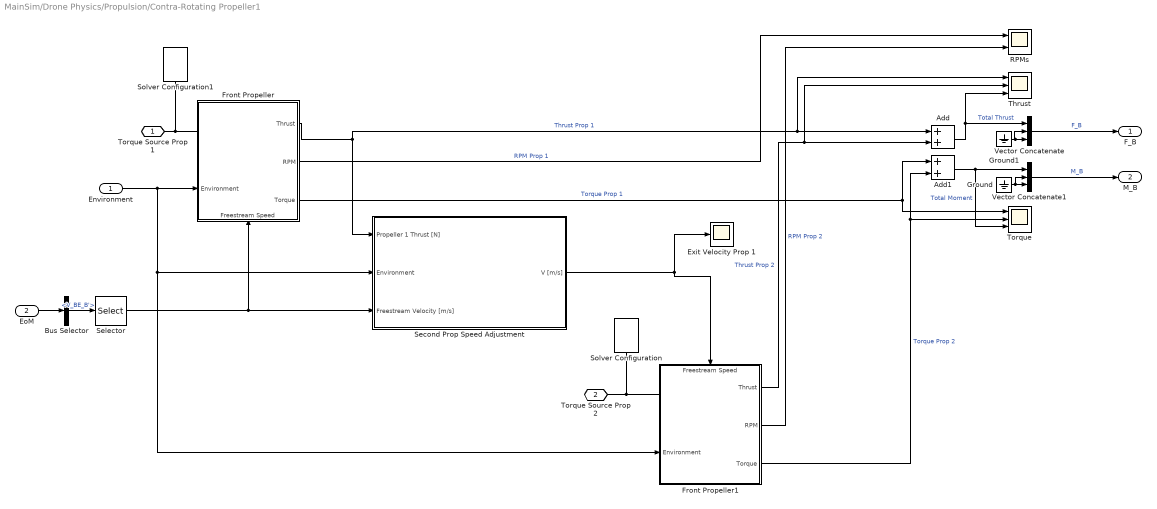
== system MainSim/Drone Physics/Propulsion/Contra-Rotating Propeller1 ==
  Environment : Inport
  EoM : Inport  Port=2
  Add : Sum
  Add1 : Sum
  Bus Selector : BusSelector  OutputSignals=V_BE_B'
  Exit Velocity Prop 1 : Scope
      settings: ActiveDisplayYMinimum=8.9336789456286088  ActiveDisplayYMaximum=11.068772464025542  DataLoggingVariableName=ScopeData5
  Front Propeller : Subsystem
      settings: PortSchema="{\"entries\":[{\"content\":{\"sides\":[{\"content\":{\"connectorIds\":[\"LConn1\",\"In1\"]},\"type\":\"ConnectorPlacement.EquallySpacedRectSide\",\"uuid\":\"73d37dfa-c503-43f9-9596-b5e45f2bb291\"},{\"content\":{\"connectorIds\":[\"Out1\",\"Out2\",\"Out3\"],\"side\":\"RIGHT\"},\"type\":\"ConnectorPlacement.EquallySpacedRectSide\",\"uuid\":\"3674c389-2fff-4609-bdea-497312b626f0\"},{\"content\":{\"side\":\"TOP\"},\"type\":\"ConnectorPlacement.EquallySpacedRectSide\",\"uuid\":\"4ddff869-abc5-41ea-b654-b1a87db3aebf\"},{\"content\":{\"connectorIds\":[\"In2\"],\"side\":\"BOTTOM\"},\"type\":\"ConnectorPlacement.EquallySpacedRectSide\",\"uuid\":\"b118b9bb-d518-4709-95e5-457ee8be32dc\"}]},\"type\":\"ConnectorPlacement.EquallySpacedConnector\",\"uuid\":\"ef4d0754-f307-49aa-90cb-f59c4d3f0201\"}],\"packageUris\":[\"http://schema.mathworks.com/mf0/Connector/R2020b\"],\"version\":\"1.0\"}"
  Front Propeller1 : Subsystem
      settings: PortSchema="{\"entries\":[{\"content\":{\"sides\":[{\"content\":{\"connectorIds\":[\"LConn1\",\"In1\"]},\"type\":\"ConnectorPlacement.EquallySpacedRectSide\",\"uuid\":\"73d37dfa-c503-43f9-9596-b5e45f2bb291\"},{\"content\":{\"connectorIds\":[\"Out1\",\"Out2\",\"Out3\"],\"side\":\"RIGHT\"},\"type\":\"ConnectorPlacement.EquallySpacedRectSide\",\"uuid\":\"3674c389-2fff-4609-bdea-497312b626f0\"},{\"content\":{\"connectorIds\":[\"In2\"],\"side\":\"TOP\"},\"type\":\"ConnectorPlacement.EquallySpacedRectSide\",\"uuid\":\"4ddff869-abc5-41ea-b654-b1a87db3aebf\"}]},\"type\":\"ConnectorPlacement.EquallySpacedConnector\",\"uuid\":\"ef4d0754-f307-49aa-90cb-f59c4d3f0201\"}],\"packageUris\":[\"http://schema.mathworks.com/mf0/Connector/R2020b\"],\"version\":\"1.0\"}"
  Ground : Ground
  Ground1 : Ground
  RPMs : Scope  NumInputPorts=2
      settings: ActiveDisplayYMinimum=-11573.712044991189  ActiveDisplayYMaximum=11896.938453382989  DataLoggingVariableName=ScopeData4
  Second Prop Speed Adjustment : Subsystem
  Selector : Selector  InputPortWidth=3  IndexOptions=Index vector (dialog)  Indices=[1]  OutputSizes=1
  Solver Configuration : nesl_utility/Solver Configuration  PhysicalDomain=network_engine_domain  SubClassName=solver  LeftPortType=input  RightPortType=generic  Tones=[]  Harmonics=[]  SimulateNoise=off  Profile=off  UseLocalSampling=off  EnableSwitchedLinearOptims=on  FrequencyDomain=off  UseCCode=off  RelTol=0.001  AbsTol=0.001  MinStep=1e-09  ToWorkspace=off  RevertToSquareIcSolve=off  NumHomotopyIterations=100  PhasorMode=off  PhasorModeNumHarmonics=1  ConsistencySolver=NEWTON_XTOL_AFTER_FTOL  IndexReductionMethod=DerivativeReplacement  DoDC=off  ResidualTolerance=1e-09  ConsistencyTolSource=GLOBAL  ConsistencyAbsTol=0.001  ConsistencyRelTol=0.001  ConsistencyTolFactor=0.001  UseLocalSolver=off  LocalSolverChoice=NE_BACKWARD_EULER_ADVANCER  ResolveIndetEquations=on  FunctionEvalNumThread=1  LocalSolverSampleTime=0.001  DoFixedCost=off  MaxNonlinIter=3  MaxModeIter=2  ComputeImpulses=off  ImpulseIterations=2  LinearAlgebra=auto  LinearAlgebraNumThread=0  EquationFormulation=NE_TIME_EF  DelaysMemoryBudget=1024  AutomaticFiltering=on  FilteringTimeConstant=0.001  PartitionStorageMethod=AS_NEEDED  PartitionMemoryBudget=1024  PartitionMethod=ROBUST  MultibodyUseLocalSolver=off  MultibodyLocalSolverChoice=ODE1  MultibodyLocalSolverSampleTime=0.001
  Solver Configuration1 : nesl_utility/Solver Configuration  PhysicalDomain=network_engine_domain  SubClassName=solver  LeftPortType=input  RightPortType=generic  Tones=[]  Harmonics=[]  SimulateNoise=off  Profile=off  UseLocalSampling=off  EnableSwitchedLinearOptims=on  FrequencyDomain=off  UseCCode=off  RelTol=0.001  AbsTol=0.001  MinStep=1e-09  ToWorkspace=off  RevertToSquareIcSolve=off  NumHomotopyIterations=100  PhasorMode=off  PhasorModeNumHarmonics=1  ConsistencySolver=NEWTON_XTOL_AFTER_FTOL  IndexReductionMethod=DerivativeReplacement  DoDC=off  ResidualTolerance=1e-09  ConsistencyTolSource=GLOBAL  ConsistencyAbsTol=0.001  ConsistencyRelTol=0.001  ConsistencyTolFactor=0.001  UseLocalSolver=off  LocalSolverChoice=NE_BACKWARD_EULER_ADVANCER  ResolveIndetEquations=on  FunctionEvalNumThread=1  LocalSolverSampleTime=0.001  DoFixedCost=off  MaxNonlinIter=3  MaxModeIter=2  ComputeImpulses=off  ImpulseIterations=2  LinearAlgebra=auto  LinearAlgebraNumThread=0  EquationFormulation=NE_TIME_EF  DelaysMemoryBudget=1024  AutomaticFiltering=on  FilteringTimeConstant=0.001  PartitionStorageMethod=AS_NEEDED  PartitionMemoryBudget=1024  PartitionMethod=ROBUST  MultibodyUseLocalSolver=off  MultibodyLocalSolverChoice=ODE1  MultibodyLocalSolverSampleTime=0.001
  Thrust : Scope  NumInputPorts=3
      settings: ActiveDisplayYMinimum=0.33826860057429142  ActiveDisplayYMaximum=0.39208387213902191
  Torque : Scope  NumInputPorts=3
      settings: ActiveDisplayYMinimum=-0.01855336181218363  ActiveDisplayYMaximum=0.018553497462872586  DataLoggingVariableName=ScopeData6
  Vector Concatenate : Concatenate  NumInputs=3
  Vector Concatenate1 : Concatenate  NumInputs=3
  Torque Source Prop 1 : PMIOPort  Side=Left
  Torque Source Prop 2 : PMIOPort  Port=2  Side=Left
  F_B : Outport
  M_B : Outport  Port=2
  wires:
  Add/1 -> Thrust/3, Vector Concatenate/1  "Total Thrust"
  Selector/1 -> Front Propeller/2(Freestream Speed), Second Prop Speed Adjustment/3(Freestream Velocity [m/s])
  Ground/1 -> Vector Concatenate1/2, Vector Concatenate1/3
  Vector Concatenate/1 -> F_B/1  "F_B"
  Front Propeller1/1(Thrust) -> Thrust/2, Add/2  "Thrust Prop 2"
  Front Propeller/3(Torque) -> Torque/1, Add1/1  "Torque Prop 1"
  Ground1/1 -> Vector Concatenate/2, Vector Concatenate/3
  Front Propeller1/3(Torque) -> Add1/2, Torque/2  "Torque Prop 2"
  Front Propeller1/2(RPM) -> RPMs/2  "RPM Prop 2"
  Vector Concatenate1/1 -> M_B/1  "M_B"
  Environment/1 -> Front Propeller1/1(Environment), Second Prop Speed Adjustment/2(Environment), Front Propeller/1(Environment)
  Front Propeller/2(RPM) -> RPMs/1  "RPM Prop 1"
  Second Prop Speed Adjustment/1(V [m/s]) -> Front Propeller1/2(Freestream Speed), Exit Velocity Prop 1/1
  Add1/1 -> Torque/3, Vector Concatenate1/1  "Total Moment"
  Front Propeller/1(Thrust) -> Thrust/1, Add/1, Second Prop Speed Adjustment/1(Propeller 1 Thrust [N])  "Thrust Prop 1"
  EoM/1 -> Bus Selector/1
  Bus Selector/1 -> Selector/1  "<V_BE_B'>"
  connections:
  Torque Source Prop 2/RConn1 -- Front Propeller1/LConn1 -- Solver Configuration/RConn1
  Torque Source Prop 1/RConn1 -- Solver Configuration1/RConn1 -- Front Propeller/LConn1

== system MainSim/Drone Physics/Propulsion/ESC and Motor ==
  Input Motor 1 : Inport
  Input Motor 2 : Inport  Port=2
  Gain : Gain  Gain=-1
  Gain1 : Gain
  Ideal Angular Velocity Source : fl_lib/Mechanical/Mechanical Sources/Ideal Angular Velocity Source
  Ideal Angular Velocity Source1 : fl_lib/Mechanical/Mechanical Sources/Ideal Angular Velocity Source
  Mechanical Rotational Reference : fl_lib/Mechanical/Rotational Elements/Mechanical Rotational Reference
  Mechanical Rotational Reference1 : fl_lib/Mechanical/Rotational Elements/Mechanical Rotational Reference
  Scope : Scope  NumInputPorts=2
      settings: ActiveDisplayYMinimum=-1  ActiveDisplayYMaximum=1  DataLoggingVariableName=ScopeData11
  Simulink-PS Converter : nesl_utility/Simulink-PS Converter  PhysicalDomain=network_engine_domain  SubClassName=ps_input  LeftPortType=input  RightPortType=output  PseudoPeriodic=off  Frequencies=[]  NoiseDistribution=none  NoiseParameters=[]  Unit=rad/s  AffineConversion=off  FilteringAndDerivatives=filter  SimscapeFilterOrder=1  InputFilterTimeConstant=0.001  UdotUserProvided=0
  Simulink-PS Converter1 : nesl_utility/Simulink-PS Converter  PhysicalDomain=network_engine_domain  SubClassName=ps_input  LeftPortType=input  RightPortType=output  PseudoPeriodic=off  Frequencies=[]  NoiseDistribution=none  NoiseParameters=[]  Unit=rad/s  AffineConversion=off  FilteringAndDerivatives=filter  SimscapeFilterOrder=1  InputFilterTimeConstant=0.001  UdotUserProvided=0
  Transfer Fcn : TransferFcn  Numerator=[1000]  Denominator=[1/20 1]
  Transfer Fcn1 : TransferFcn  Numerator=[1000]  Denominator=[1/20 1]
  Motor 1 : PMIOPort  Side=Right
  Motor 2 : PMIOPort  Port=2  Side=Right
  wires:
  Gain/1 -> Scope/2, Simulink-PS Converter1/1
  Transfer Fcn/1 -> Scope/1, Simulink-PS Converter/1
  Input Motor 2/1 -> Transfer Fcn1/1
  Input Motor 1/1 -> Gain1/1
  Transfer Fcn1/1 -> Gain/1
  Gain1/1 -> Transfer Fcn/1
  connections:
  Ideal Angular Velocity Source1/LConn1 -- Motor 2/RConn1
  Ideal Angular Velocity Source/RConn1 -- Simulink-PS Converter/RConn1
  Ideal Angular Velocity Source/LConn1 -- Motor 1/RConn1
  Mechanical Rotational Reference/LConn1 -- Ideal Angular Velocity Source/RConn2
  Mechanical Rotational Reference1/LConn1 -- Ideal Angular Velocity Source1/RConn2
  Ideal Angular Velocity Source1/RConn1 -- Simulink-PS Converter1/RConn1

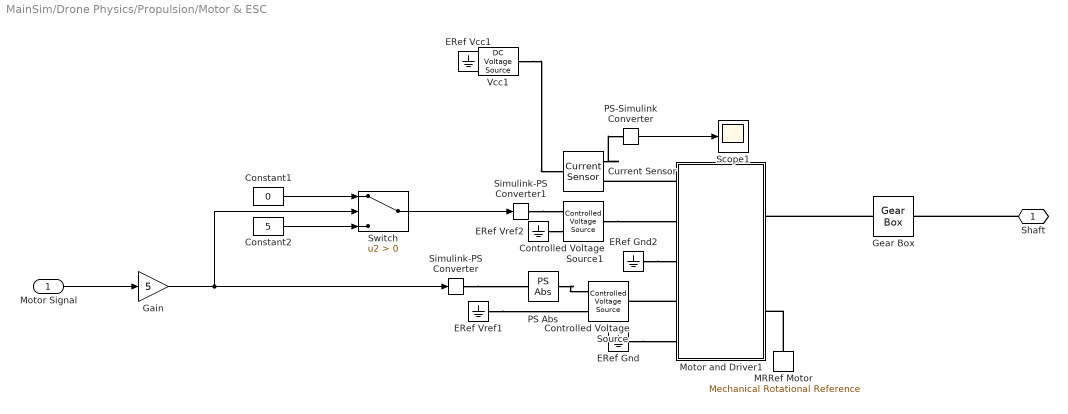
== system MainSim/Drone Physics/Propulsion/Motor & ESC ==
  Motor Signal : Inport
  Constant1 : Constant  Value=0
  Constant2 : Constant  Value=5
  Controlled Voltage Source : fl_lib/Electrical/Electrical Sources/Controlled Voltage Source
  Controlled Voltage Source1 : fl_lib/Electrical/Electrical Sources/Controlled Voltage Source
  Current Sensor : fl_lib/Electrical/Electrical Sensors/Current Sensor
  ERef Vcc1 : fl_lib/Electrical/Electrical Elements/Electrical Reference
  ERef Vref1 : fl_lib/Electrical/Electrical Elements/Electrical Reference
  ERef Vref2 : fl_lib/Electrical/Electrical Elements/Electrical Reference
  ERef Gnd : fl_lib/Electrical/Electrical Elements/Electrical Reference
  ERef Gnd2 : fl_lib/Electrical/Electrical Elements/Electrical Reference
  Gain : Gain  Gain=5
  Gear Box : fl_lib/Mechanical/Mechanisms/Gear Box  ratio=-1  t_in_specify=off  t_in_priority=None  t_in=0 N*m  t_in_nominal_specify=off  t_in_nominal_value=1  t_in_nominal_unit=N*m  t_out_specify=off  t_out_priority=None  t_out=0 N*m  t_out_nominal_specify=off  t_out_nominal_value=1  t_out_nominal_unit=N*m
  MRRef Motor : fl_lib/Mechanical/Rotational Elements/Mechanical Rotational Reference
  Motor and Driver1 : Subsystem  Tag=PublishSubsystem  mask(Servomotor & Driver){Vcc=7.4, I0=0.54, T_i=0.005, eta=65, rpm_eta=18000, trq_eta=0.02, trq_stall=0.0685, Kp=0.00002, Ki=0.000004, Vref_max=5, rpm_max=16243, J=2*1e-7, rpm0=0}
      mask prompts: Vcc "Nominal voltage (V)"; I0 "No-load DC current to driver (A)"; T_i "Current loop time constant (s)"; eta "Efficiency (%)"; rpm_eta "Speed at which efficiency measured (rpm)"; trq_eta "Torque at which efficiency measured  (Nm)"; trq_stall "Stall torque (Nm)"; Kp "Proportional gain"; Ki "Integral gain"; Vref_max "Maximum reference voltage (V)"; rpm_max "Speed at maximum reference voltage (rpm)"; J "Rotor inerita (kg*m^2)"; rpm0 "Rotor initial speed (rpm)"
      mask help: Implements an abstracted model of a servomotor and driver configured for closed-loop speed control.
  PS Abs : fl_lib/Physical Signals/Nonlinear Operators/PS Abs  ZeroCross=true
      settings: InternalSimscapePortConfiguration="{\"Bottom\":[],\"Left\":[{\"id\":\"I\",\"label\":\"\",\"type\":\"input\"}],\"Right\":[{\"id\":\"O\",\"label\":\"\",\"type\":\"output\"}],\"Top\":[]}"
  PS-Simulink Converter : nesl_utility/PS-Simulink Converter  PhysicalDomain=network_engine_domain  SubClassName=ps_output  LeftPortType=input  RightPortType=output  PseudoPeriodic=off  Frequencies=[]  VectorFormat=inherit  Unit=inherit  AffineConversion=off
  Scope1 : Scope
      settings: ActiveDisplayYMinimum=-1.7935370695604353  ActiveDisplayYMaximum=9.025093295510743
  Simulink-PS Converter : nesl_utility/Simulink-PS Converter  PhysicalDomain=network_engine_domain  SubClassName=ps_input  LeftPortType=input  RightPortType=output  PseudoPeriodic=off  Frequencies=[]  NoiseDistribution=none  NoiseParameters=[]  Unit=1  AffineConversion=off  FilteringAndDerivatives=provide  SimscapeFilterOrder=1  InputFilterTimeConstant=0.001  UdotUserProvided=0
  Simulink-PS Converter1 : nesl_utility/Simulink-PS Converter  PhysicalDomain=network_engine_domain  SubClassName=ps_input  LeftPortType=input  RightPortType=output  PseudoPeriodic=off  Frequencies=[]  NoiseDistribution=none  NoiseParameters=[]  Unit=1  AffineConversion=off  FilteringAndDerivatives=provide  SimscapeFilterOrder=1  InputFilterTimeConstant=0.001  UdotUserProvided=0
  Switch : Switch  Criteria=u2 > Threshold  SaturateOnIntegerOverflow=off  InputSameDT=off
  Vcc1 : fl_lib/Electrical/Electrical Sources/DC Voltage Source  v0=14.8/2 V
      settings: AttributesFormatString=%<v0> %<v0_unit>
  Shaft : PMIOPort  Side=Right
  wires:
  Switch/1 -> Simulink-PS Converter1/1
  Motor Signal/1 -> Gain/1
  PS-Simulink Converter/1 -> Scope1/1
  Gain/1 -> Switch/2, Simulink-PS Converter/1
  Constant1/1 -> Switch/1
  Constant2/1 -> Switch/3
  connections:
  Gear Box/LConn1 -- Motor and Driver1/RConn1
  ERef Vref2/LConn1 -- Controlled Voltage Source1/RConn2
  Controlled Voltage Source1/LConn1 -- Motor and Driver1/LConn2
  Motor and Driver1/LConn1 -- Current Sensor/RConn2
  Simulink-PS Converter/RConn1 -- PS Abs/LConn1
  MRRef Motor/LConn1 -- Motor and Driver1/RConn2
  ERef Gnd2/LConn1 -- Motor and Driver1/LConn3
  ERef Gnd/LConn1 -- Motor and Driver1/LConn5
  ERef Vref1/LConn1 -- Controlled Voltage Source/RConn2
  Vcc1/LConn1 -- Current Sensor/LConn1
  PS Abs/RConn1 -- Controlled Voltage Source/RConn1
  Motor and Driver1/LConn4 -- Controlled Voltage Source/LConn1
  ERef Vcc1/LConn1 -- Vcc1/RConn1
  Simulink-PS Converter1/RConn1 -- Controlled Voltage Source1/RConn1
  Current Sensor/RConn1 -- PS-Simulink Converter/LConn1
  Shaft/RConn1 -- Gear Box/RConn1

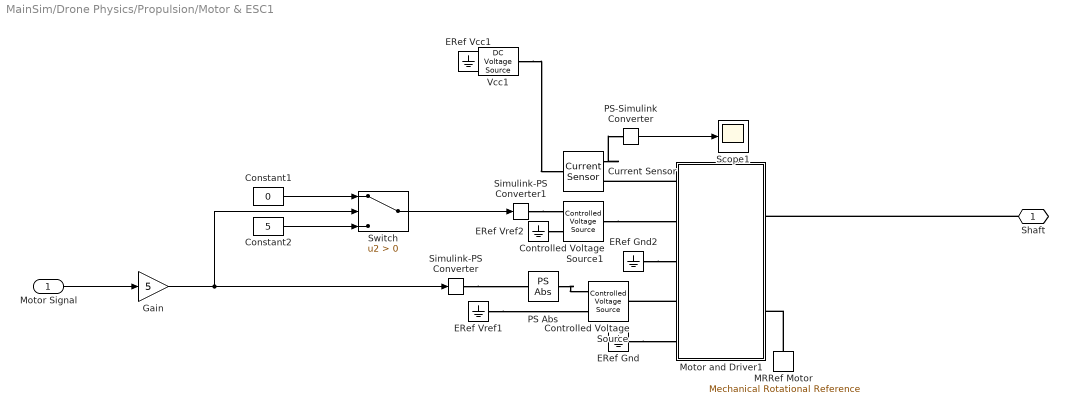
== system MainSim/Drone Physics/Propulsion/Motor & ESC1 ==
  Motor Signal : Inport
  Constant1 : Constant  Value=0
  Constant2 : Constant  Value=5
  Controlled Voltage Source : fl_lib/Electrical/Electrical Sources/Controlled Voltage Source
  Controlled Voltage Source1 : fl_lib/Electrical/Electrical Sources/Controlled Voltage Source
  Current Sensor : fl_lib/Electrical/Electrical Sensors/Current Sensor
  ERef Vcc1 : fl_lib/Electrical/Electrical Elements/Electrical Reference
  ERef Vref1 : fl_lib/Electrical/Electrical Elements/Electrical Reference
  ERef Vref2 : fl_lib/Electrical/Electrical Elements/Electrical Reference
  ERef Gnd : fl_lib/Electrical/Electrical Elements/Electrical Reference
  ERef Gnd2 : fl_lib/Electrical/Electrical Elements/Electrical Reference
  Gain : Gain  Gain=5
  MRRef Motor : fl_lib/Mechanical/Rotational Elements/Mechanical Rotational Reference
  Motor and Driver1 : Subsystem  Tag=PublishSubsystem  mask(Servomotor & Driver){Vcc=7.4, I0=0.54, T_i=0.005, eta=65, rpm_eta=18000, trq_eta=0.02, trq_stall=0.0685, Kp=0.00002, Ki=0.000004, Vref_max=5, rpm_max=16243, J=2*1e-7, rpm0=0}
      mask prompts: Vcc "Nominal voltage (V)"; I0 "No-load DC current to driver (A)"; T_i "Current loop time constant (s)"; eta "Efficiency (%)"; rpm_eta "Speed at which efficiency measured (rpm)"; trq_eta "Torque at which efficiency measured  (Nm)"; trq_stall "Stall torque (Nm)"; Kp "Proportional gain"; Ki "Integral gain"; Vref_max "Maximum reference voltage (V)"; rpm_max "Speed at maximum reference voltage (rpm)"; J "Rotor inerita (kg*m^2)"; rpm0 "Rotor initial speed (rpm)"
      mask help: Implements an abstracted model of a servomotor and driver configured for closed-loop speed control.
  PS Abs : fl_lib/Physical Signals/Nonlinear Operators/PS Abs  ZeroCross=true
      settings: InternalSimscapePortConfiguration="{\"Bottom\":[],\"Left\":[{\"id\":\"I\",\"label\":\"\",\"type\":\"input\"}],\"Right\":[{\"id\":\"O\",\"label\":\"\",\"type\":\"output\"}],\"Top\":[]}"
  PS-Simulink Converter : nesl_utility/PS-Simulink Converter  PhysicalDomain=network_engine_domain  SubClassName=ps_output  LeftPortType=input  RightPortType=output  PseudoPeriodic=off  Frequencies=[]  VectorFormat=inherit  Unit=inherit  AffineConversion=off
  Scope1 : Scope
      settings: ActiveDisplayYMinimum=-1.7935370695604353  ActiveDisplayYMaximum=9.025093295510743
  Simulink-PS Converter : nesl_utility/Simulink-PS Converter  PhysicalDomain=network_engine_domain  SubClassName=ps_input  LeftPortType=input  RightPortType=output  PseudoPeriodic=off  Frequencies=[]  NoiseDistribution=none  NoiseParameters=[]  Unit=1  AffineConversion=off  FilteringAndDerivatives=provide  SimscapeFilterOrder=1  InputFilterTimeConstant=0.001  UdotUserProvided=0
  Simulink-PS Converter1 : nesl_utility/Simulink-PS Converter  PhysicalDomain=network_engine_domain  SubClassName=ps_input  LeftPortType=input  RightPortType=output  PseudoPeriodic=off  Frequencies=[]  NoiseDistribution=none  NoiseParameters=[]  Unit=1  AffineConversion=off  FilteringAndDerivatives=provide  SimscapeFilterOrder=1  InputFilterTimeConstant=0.001  UdotUserProvided=0
  Switch : Switch  Criteria=u2 > Threshold  SaturateOnIntegerOverflow=off  InputSameDT=off
  Vcc1 : fl_lib/Electrical/Electrical Sources/DC Voltage Source  v0=14.8/2 V
      settings: AttributesFormatString=%<v0> %<v0_unit>
  Shaft : PMIOPort  Side=Right
  wires:
  Switch/1 -> Simulink-PS Converter1/1
  Motor Signal/1 -> Gain/1
  PS-Simulink Converter/1 -> Scope1/1
  Gain/1 -> Switch/2, Simulink-PS Converter/1
  Constant1/1 -> Switch/1
  Constant2/1 -> Switch/3
  connections:
  Shaft/RConn1 -- Motor and Driver1/RConn1
  ERef Vref2/LConn1 -- Controlled Voltage Source1/RConn2
  Controlled Voltage Source1/LConn1 -- Motor and Driver1/LConn2
  Motor and Driver1/LConn1 -- Current Sensor/RConn2
  Simulink-PS Converter/RConn1 -- PS Abs/LConn1
  MRRef Motor/LConn1 -- Motor and Driver1/RConn2
  ERef Gnd2/LConn1 -- Motor and Driver1/LConn3
  ERef Gnd/LConn1 -- Motor and Driver1/LConn5
  ERef Vref1/LConn1 -- Controlled Voltage Source/RConn2
  Vcc1/LConn1 -- Current Sensor/LConn1
  PS Abs/RConn1 -- Controlled Voltage Source/RConn1
  Motor and Driver1/LConn4 -- Controlled Voltage Source/LConn1
  ERef Vcc1/LConn1 -- Vcc1/RConn1
  Simulink-PS Converter1/RConn1 -- Controlled Voltage Source1/RConn1
  Current Sensor/RConn1 -- PS-Simulink Converter/LConn1
